simulink model "slab02"  (R2023b)
settings: Solver=VariableStepAuto  StartTime=0.0  StopTime=20  RelTol=1e-3
values from neighbouring files (symbols this model uses):
  C = [1 0 0]    [lab3.m]
undefined symbols (not defined in the file or in its folder): fg1_chua, ga, mu_chua, ref_chua, u_chua
settings Model: Creator=s331564  LastModifiedBy=luigi

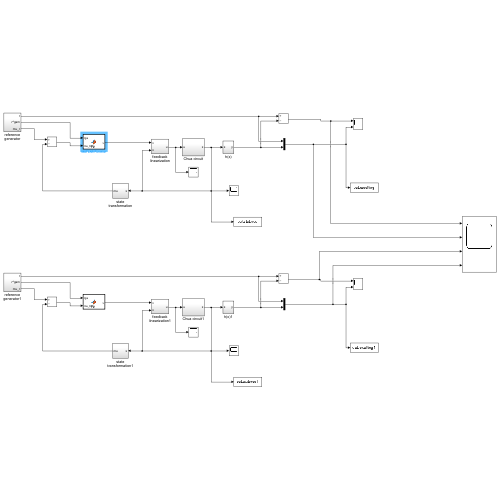
[thumbnail: Simulink's stored preview of the top-level diagram]
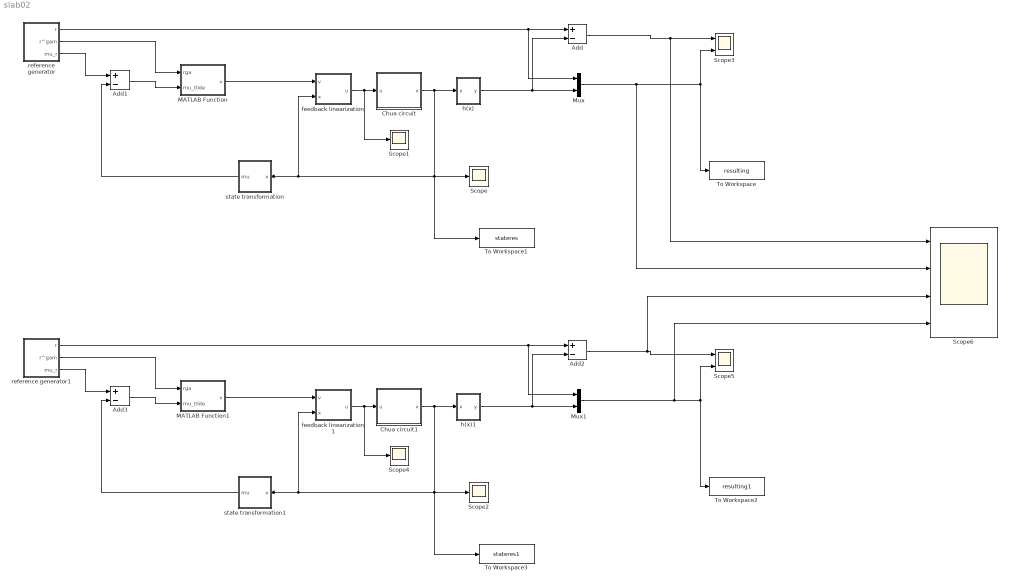
== system slab02 ==
  Add{,1..3} (4 alike) : Sum  Inputs=+-
  Chua circuit : Subsystem
  Chua circuit1 : Subsystem
  MATLAB Function : MATLAB Function  TreatAsAtomicUnit=on
  MATLAB Function1 : MATLAB Function  TreatAsAtomicUnit=on
  Mux : Mux  Inputs=2
  Mux1 : Mux  Inputs=2
  Scope{,1..2,4} (4 alike) : Scope
  Scope3 : Scope  NumInputPorts=2
  Scope5 : Scope  NumInputPorts=2
  Scope6 : Scope  NumInputPorts=4
  To Workspace : ToWorkspace  VariableName=resulting  SaveFormat=Timeseries  SampleTime=-1
  To Workspace1 : ToWorkspace  VariableName=stateres  SaveFormat=Timeseries  SampleTime=-1
  To Workspace2 : ToWorkspace  VariableName=resulting1  SaveFormat=Timeseries  SampleTime=-1
  To Workspace3 : ToWorkspace  VariableName=stateres1  SaveFormat=Timeseries  SampleTime=-1
  feedback linearization : Subsystem
  feedback linearization1 : Subsystem
  h(x) : Subsystem
  h(x)1 : Subsystem
  reference generator : Subsystem
  reference generator1 : Subsystem
  state transformation : Subsystem
  state transformation1 : Subsystem
  wires:
  MATLAB Function/1(v) -> feedback linearization/1(v)
  state transformation/1(mu) -> Add1/2
  Add1/1 -> MATLAB Function/2(mu_tilde)
  reference generator/2(r^gam) -> MATLAB Function/1(rga)
  Add/1 -> Scope6/1, Scope3/1
  h(x)/1(y) -> Add/2, Mux/2
  reference generator/1(r) -> Mux/1, Add/1
  Chua circuit/1(x) -> h(x)/1(x), To Workspace1/1, feedback linearization/2(x), state transformation/1(x), Scope/1
  reference generator/3(mu_r) -> Add1/1
  Mux/1 -> Scope6/2, Scope3/2, To Workspace/1
  feedback linearization/1(u) -> Scope1/1, Chua circuit/1(u)
  feedback linearization1/1(u) -> Scope4/1, Chua circuit1/1(u)
  h(x)1/1(y) -> Add2/2, Mux1/2
  Mux1/1 -> Scope6/4, Scope5/2, To Workspace2/1
  Add3/1 -> MATLAB Function1/2(mu_tilde)
  MATLAB Function1/1(v) -> feedback linearization1/1(v)
  state transformation1/1(mu) -> Add3/2
  reference generator1/1(r) -> Mux1/1, Add2/1
  Add2/1 -> Scope6/3, Scope5/1
  reference generator1/3(mu_r) -> Add3/1
  Chua circuit1/1(x) -> h(x)1/1(x), To Workspace3/1, feedback linearization1/2(x), state transformation1/1(x), Scope2/1
  reference generator1/2(r^gam) -> MATLAB Function1/1(rga)

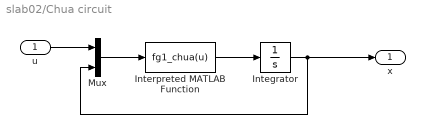
== system slab02/Chua circuit ==
  u : Inport
  Integrator : Integrator  InitialCondition=[0; 0; 0]
  Interpreted MATLAB Function : MATLABFcn  MATLABFcn=fg1_chua(u)
  Mux : Mux  Inputs=2
  x : Outport  VectorParamsAs1DForOutWhenUnconnected=off
  wires:
  u/1 -> Mux/1
  Interpreted MATLAB Function/1 -> Integrator/1
  Integrator/1 -> Mux/2, x/1
  Mux/1 -> Interpreted MATLAB Function/1

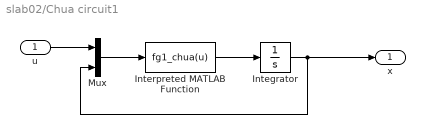
== system slab02/Chua circuit1 ==
  u : Inport
  Integrator : Integrator  InitialCondition=[0; 0; 0]
  Interpreted MATLAB Function : MATLABFcn  MATLABFcn=fg1_chua(u)
  Mux : Mux  Inputs=2
  x : Outport  VectorParamsAs1DForOutWhenUnconnected=off
  wires:
  u/1 -> Mux/1
  Interpreted MATLAB Function/1 -> Integrator/1
  Integrator/1 -> Mux/2, x/1
  Mux/1 -> Interpreted MATLAB Function/1

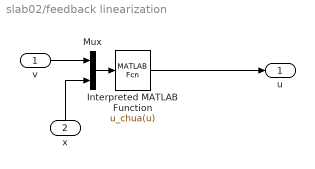
== system slab02/feedback linearization ==
  v : Inport
  x : Inport  Port=2
  Interpreted MATLAB Function : MATLABFcn  MATLABFcn=u_chua(u)  OutputSignalType=real
  Mux : Mux  Inputs=2
  u : Outport  VectorParamsAs1DForOutWhenUnconnected=off
  wires:
  x/1 -> Mux/2
  Mux/1 -> Interpreted MATLAB Function/1
  v/1 -> Mux/1
  Interpreted MATLAB Function/1 -> u/1

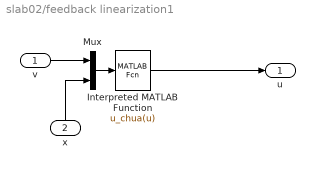
== system slab02/feedback linearization1 ==
  v : Inport
  x : Inport  Port=2
  Interpreted MATLAB Function : MATLABFcn  MATLABFcn=u_chua(u)  OutputSignalType=real
  Mux : Mux  Inputs=2
  u : Outport  VectorParamsAs1DForOutWhenUnconnected=off
  wires:
  x/1 -> Mux/2
  Mux/1 -> Interpreted MATLAB Function/1
  v/1 -> Mux/1
  Interpreted MATLAB Function/1 -> u/1

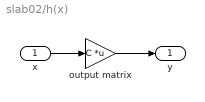
== system slab02/h(x) ==
  x : Inport
  output matrix : Gain  Gain=C  Multiplication=Matrix(K*u)
  y : Outport  VectorParamsAs1DForOutWhenUnconnected=off
  wires:
  x/1 -> output matrix/1
  output matrix/1 -> y/1

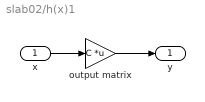
== system slab02/h(x)1 ==
  x : Inport
  output matrix : Gain  Gain=C  Multiplication=Matrix(K*u)
  y : Outport  VectorParamsAs1DForOutWhenUnconnected=off
  wires:
  x/1 -> output matrix/1
  output matrix/1 -> y/1

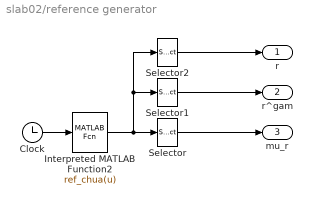
== system slab02/reference generator ==
  Clock : Clock
  Interpreted MATLAB Function2 : MATLABFcn  MATLABFcn=ref_chua(u)
  Selector : Selector  InputPortWidth=ga+1  IndexOptions=Index vector (dialog)  Indices=1:ga  OutputSizes=1
  Selector1 : Selector  InputPortWidth=ga+1  IndexOptions=Index vector (dialog)  Indices=ga+1  OutputSizes=1
  Selector2 : Selector  InputPortWidth=ga+1  IndexOptions=Index vector (dialog)  Indices=1  OutputSizes=1
  r : Outport  VectorParamsAs1DForOutWhenUnconnected=off
  r^gam : Outport  Port=2  VectorParamsAs1DForOutWhenUnconnected=off
  mu_r : Outport  Port=3  VectorParamsAs1DForOutWhenUnconnected=off
  wires:
  Clock/1 -> Interpreted MATLAB Function2/1
  Selector1/1 -> r^gam/1
  Selector2/1 -> r/1
  Interpreted MATLAB Function2/1 -> Selector2/1, Selector1/1, Selector/1
  Selector/1 -> mu_r/1

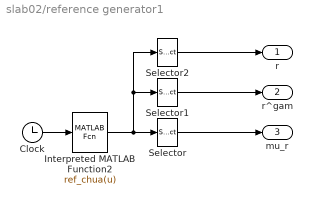
== system slab02/reference generator1 ==
  Clock : Clock
  Interpreted MATLAB Function2 : MATLABFcn  MATLABFcn=ref_chua(u)
  Selector : Selector  InputPortWidth=ga+1  IndexOptions=Index vector (dialog)  Indices=1:ga  OutputSizes=1
  Selector1 : Selector  InputPortWidth=ga+1  IndexOptions=Index vector (dialog)  Indices=ga+1  OutputSizes=1
  Selector2 : Selector  InputPortWidth=ga+1  IndexOptions=Index vector (dialog)  Indices=1  OutputSizes=1
  r : Outport  VectorParamsAs1DForOutWhenUnconnected=off
  r^gam : Outport  Port=2  VectorParamsAs1DForOutWhenUnconnected=off
  mu_r : Outport  Port=3  VectorParamsAs1DForOutWhenUnconnected=off
  wires:
  Clock/1 -> Interpreted MATLAB Function2/1
  Selector1/1 -> r^gam/1
  Selector2/1 -> r/1
  Interpreted MATLAB Function2/1 -> Selector2/1, Selector1/1, Selector/1
  Selector/1 -> mu_r/1

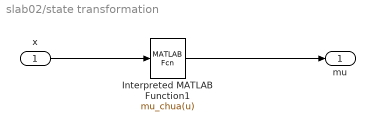
== system slab02/state transformation ==
  x : Inport
  Interpreted MATLAB Function1 : MATLABFcn  MATLABFcn=mu_chua(u)
  mu : Outport  VectorParamsAs1DForOutWhenUnconnected=off
  wires:
  x/1 -> Interpreted MATLAB Function1/1
  Interpreted MATLAB Function1/1 -> mu/1

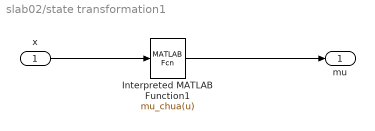
== system slab02/state transformation1 ==
  x : Inport
  Interpreted MATLAB Function1 : MATLABFcn  MATLABFcn=mu_chua(u)
  mu : Outport  VectorParamsAs1DForOutWhenUnconnected=off
  wires:
  x/1 -> Interpreted MATLAB Function1/1
  Interpreted MATLAB Function1/1 -> mu/1

== matlab function slab02/MATLAB Function ==
  data: rga input; v output; mu_tilde input
function v = fcn(rga, mu_tilde)

k2 = 30;
k1 =80;
eta = 5;
s = mu_tilde(2) + k2 * mu_tilde(1);

v = rga+ k2*mu_tilde(2)+k1*sign(eta*s);
end

== matlab function slab02/MATLAB Function1 ==
  data: rga input; v output; mu_tilde input
function v = fcn(rga, mu_tilde)

k2 = 25;
k1 = 150;

v = rga+ k2*mu_tilde(2)+k1*mu_tilde(1);
end
